simulink model "JLN_Sun_AUV_ver9"  (R2021a)
settings: Solver=VariableStepAuto  StartTime=0.0  StopTime=150  RelTol=1e-3
StopFcn:
  | figure(2)
  | plot3(Position_Data(1,1),Position_Data(1,2),Position_Data(1,3),'r*')
  | hold on
  | plot3(Position_Data(:,1),Position_Data(:,2),Position_Data(:,3));
  | plot3(Position_Data(end,1),Position_Data(end,2),Position_Data(end,3),'g*');
  | grid on
  | legend('Start Point','Trajectory','End Point')
libraries: pid_lib x4, sharedtransform x1
settings Model: Creator=logan  LastModifiedBy=naido
settings DataIOCC: ReturnWorkspaceOutputs=off

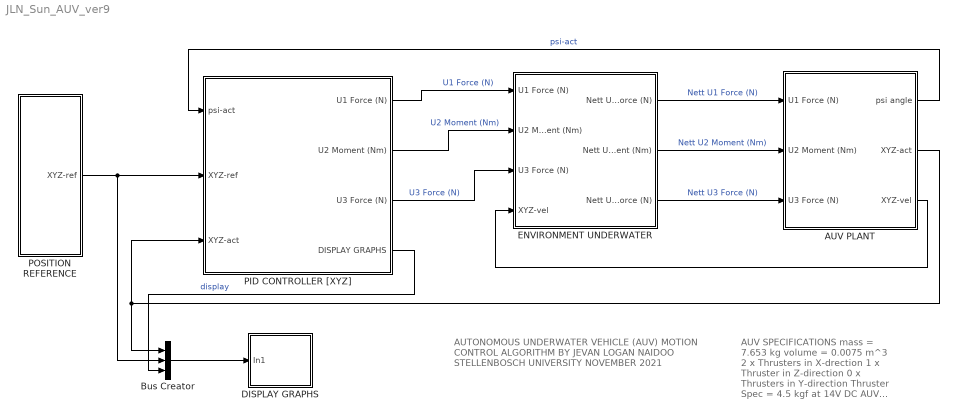
== system JLN_Sun_AUV_ver9 ==
  note: AUV SPECIFICATIONS
      | mass = 7.653 kg
      | volume = 0.0075 m^3
      | 2 x Thrusters in X-drection
      | 1 x Thruster in Z-direction
      | 0 x Thrusters in Y-direction
      | Thruster Spec = 4.5 kgf at 14V DC
      | AUV (LxWxH) = 0.500 x 0.250 x 0.150
  note: AUTONOMOUS UNDERWATER VEHICLE (AUV)
      |
      | MOTION CONTROL ALGORITHM
      | BY JEVAN LOGAN NAIDOO
      | STELLENBOSCH UNIVERSITY
      | NOVEMBER 2021
  AUV PLANT : Subsystem
  Bus Creator : BusCreator  Inputs=3
  DISPLAY GRAPHS : Subsystem
  ENVIRONMENT UNDERWATER : Subsystem
  PID CONTROLLER [XYZ] : Subsystem
  POSITION REFERENCE : Subsystem
  wires:
  AUV PLANT/1(psi angle) -> PID CONTROLLER [XYZ]/1(psi-act)  "psi-act"
  AUV PLANT/2(XYZ-act) -> PID CONTROLLER [XYZ]/3(XYZ-act), Bus Creator/1
  POSITION REFERENCE/1(XYZ-ref) -> Bus Creator/2, PID CONTROLLER [XYZ]/2(XYZ-ref)
  Bus Creator/1 -> DISPLAY GRAPHS/1(In1)
  PID CONTROLLER [XYZ]/4(DISPLAY GRAPHS) -> Bus Creator/3  "display"
  PID CONTROLLER [XYZ]/1(U1 Force (N)) -> ENVIRONMENT UNDERWATER/1(U1 Force (N))  "U1 Force (N)"
  PID CONTROLLER [XYZ]/2(U2 Moment (Nm)) -> ENVIRONMENT UNDERWATER/2(U2 Moment (Nm))  "U2 Moment (Nm)"
  PID CONTROLLER [XYZ]/3(U3 Force (N)) -> ENVIRONMENT UNDERWATER/3(U3 Force (N))  "U3 Force (N)"
  ENVIRONMENT UNDERWATER/1(Nett U1 Force (N)) -> AUV PLANT/1(U1 Force (N))  "Nett U1 Force (N)"
  ENVIRONMENT UNDERWATER/2(Nett U2 Moment (Nm)) -> AUV PLANT/2(U2 Moment (Nm))  "Nett U2 Moment (Nm)"
  ENVIRONMENT UNDERWATER/3(Nett U3 Force (N)) -> AUV PLANT/3(U3 Force (N))  "Nett U3 Force (N)"
  AUV PLANT/3(XYZ-vel) -> ENVIRONMENT UNDERWATER/4(XYZ-vel)

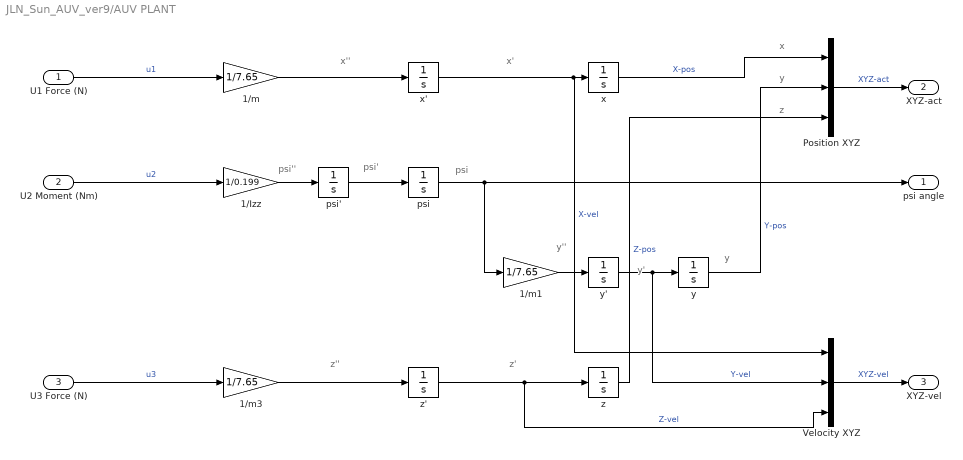
== system JLN_Sun_AUV_ver9/AUV PLANT ==
  note: z''
  note: y
  note: y'
  note: y''
  note: x
  note: psi
  note: psi'
  note: psi''
  note: x''
  note: x'
  note: z'
  note: z
  note: y
  U1 Force (N) : Inport
  U2 Moment (Nm) : Inport  Port=2
  U3 Force (N) : Inport  Port=3
  1/Izz : Gain  Gain=1/0.199
  1/m : Gain  Gain=1/7.65
  1/m1 : Gain  Gain=1/7.65
  1/m3 : Gain  Gain=1/7.65
  Position XYZ : Mux  Inputs=3
  Velocity XYZ : BusCreator  Inputs=3
  psi : Integrator
  psi' : Integrator
  x : Integrator
  x' : Integrator
  y : Integrator
  y' : Integrator
  z : Integrator
  z' : Integrator
  psi angle : Outport
  XYZ-act : Outport  Port=2
  XYZ-vel : Outport  Port=3
  wires:
  x/1 -> Position XYZ/1  "X-pos"
  y/1 -> Position XYZ/2  "Y-pos"
  U1 Force (N)/1 -> 1/m/1  "u1"
  U2 Moment (Nm)/1 -> 1/Izz/1  "u2"
  psi/1 -> 1/m1/1, psi angle/1
  psi'/1 -> psi/1
  1/Izz/1 -> psi'/1
  x'/1 -> Velocity XYZ/1, x/1  "X-vel"
  y'/1 -> Velocity XYZ/2, y/1  "Y-vel"
  1/m/1 -> x'/1
  1/m1/1 -> y'/1
  1/m3/1 -> z'/1
  z'/1 -> Velocity XYZ/3, z/1  "Z-vel"
  z/1 -> Position XYZ/3  "Z-pos"
  U3 Force (N)/1 -> 1/m3/1  "u3"
  Position XYZ/1 -> XYZ-act/1  "XYZ-act"
  Velocity XYZ/1 -> XYZ-vel/1  "XYZ-vel"

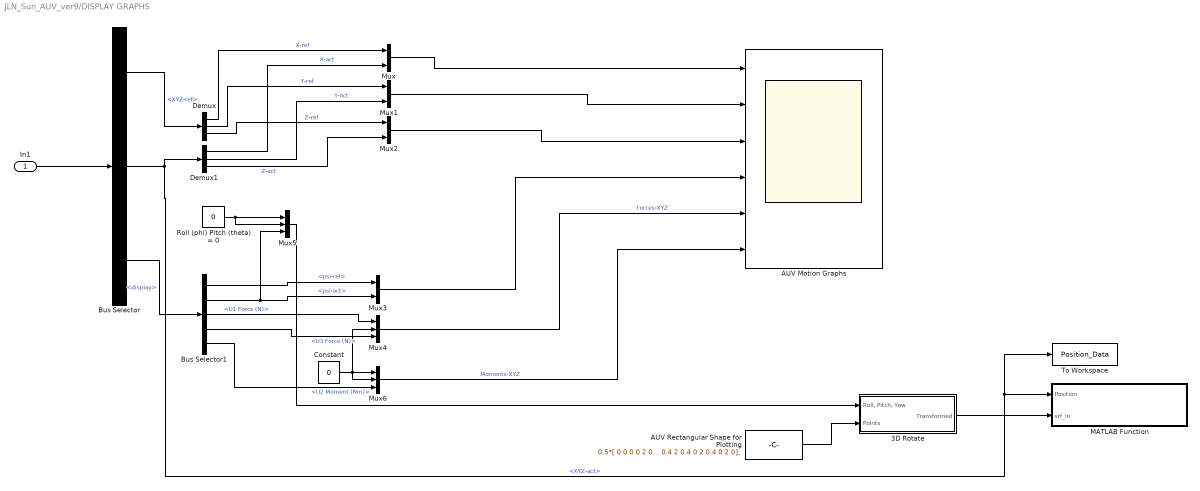
== system JLN_Sun_AUV_ver9/DISPLAY GRAPHS ==
  In1 : Inport
  "3D Rotate " : Subsystem
  AUV Motion Graphs : Scope  NumInputPorts=6
  AUV Rectangular Shape for Plotting : Constant  Value=|
      | 0.5*[	0		0		0
      | 	0		2		0
      | 	0.4		2		0
      | 	0.4		0		0
      | 	0		0		0
      | 	0		0		0.4
      | 	0		2		0.4
      | 	0.4		2		0.4
      | 	0.4		0		0.4
      | 	0		0		0.4
      | 	0.4		0		0.4
      | 	0.4		0		0
      | 	0.4		2		0
      | 	0.4		2		0.4
      | 	0		2		0.4
      | 	0		2		0];
  Bus Selector : BusSelector  OutputSignals=XYZ-ref,XYZ-act,display
  Bus Selector1 : BusSelector  OutputSignals=psi-ref,psi-act,U1 Force (N),U3 Force (N),U2 Moment (Nm)
  Constant : Constant  Value=0
  Demux : Demux  Outputs=3
  Demux1 : Demux  Outputs=3
  MATLAB Function : MATLAB Function  TreatAsAtomicUnit=on  SystemSampleTime=0.05
  Mux{,1..3} (4 alike) : Mux  Inputs=2
  Mux4 : Mux  Inputs=3
  Mux5 : Mux  Inputs=3
  Mux6 : Mux  Inputs=3
  Roll (phi) Pitch (theta) = 0 : Constant  Value=0
  To Workspace : ToWorkspace  VariableName=Position_Data  SampleTime=-1
  wires:
  Mux2/1 -> AUV Motion Graphs/3
  Mux3/1 -> AUV Motion Graphs/4
  In1/1 -> Bus Selector/1
  Mux/1 -> AUV Motion Graphs/1
  Mux1/1 -> AUV Motion Graphs/2
  Roll (phi) Pitch (theta) = 0/1 -> Mux5/1, Mux5/2
  Mux5/1 -> "3D Rotate "/1("Roll, Pitch, Yaw")
  Bus Selector/1 -> Demux/1  "<XYZ-ref>"
  Demux/1 -> Mux/1  "X-ref"
  Demux/2 -> Mux1/1  "Y-ref"
  Demux/3 -> Mux2/1  "Z-ref"
  Bus Selector/2 -> To Workspace/1, MATLAB Function/1(Position), Demux1/1  "<XYZ-act>"
  Demux1/1 -> Mux/2  "X-act"
  Demux1/2 -> Mux1/2  "Y-act"
  Demux1/3 -> Mux2/2  "Z-act"
  Bus Selector/3 -> Bus Selector1/1  "<display>"
  Bus Selector1/1 -> Mux3/1  "<psi-ref>"
  Bus Selector1/2 -> Mux5/3, Mux3/2  "<psi-act>"
  Bus Selector1/3 -> Mux4/1  "<U1 Force (N)>"
  Constant/1 -> Mux4/2, Mux6/2, Mux6/1
  Mux4/1 -> AUV Motion Graphs/5  "Forces-XYZ"
  Bus Selector1/5 -> Mux6/3  "<U2 Moment (Nm)>"
  Mux6/1 -> AUV Motion Graphs/6  "Moments-XYZ"
  Bus Selector1/4 -> Mux4/3  "<U3 Force (N)>"
  AUV Rectangular Shape for Plotting/1 -> "3D Rotate "/2(Points)
  "3D Rotate "/1("Transformed ") -> MATLAB Function/2(srf_in)

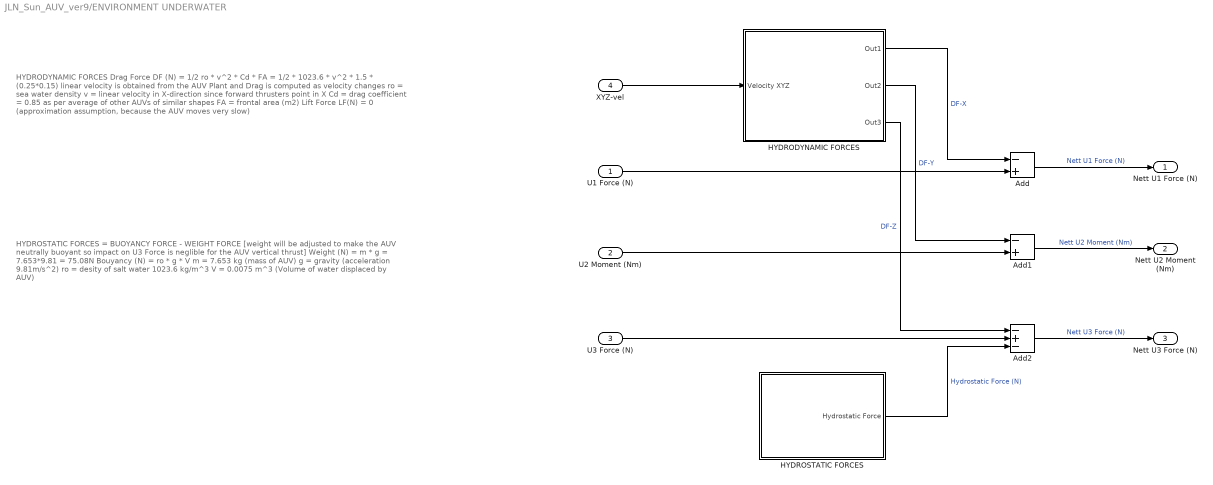
== system JLN_Sun_AUV_ver9/ENVIRONMENT UNDERWATER ==
  note: HYDRODYNAMIC FORCES
      | Drag Force DF (N) = 1/2 ro * v^2 * Cd * FA = 1/2 * 1023.6 * v^2 * 1.5 * (0.25*0.15)
      | linear velocity is obtained from the AUV Plant and Drag is computed as velocity changes
      | ro = sea water density
      | v = linear velocity in X-direction since forward thrusters point in X
      | Cd = drag coefficient = 0.85 as per average of other AUVs of similar shapes
      | FA = frontal area (m2)
      | Lift Force LF(N) = 0 (approximation assumption, because the AUV moves very slow)
  note: HYDROSTATIC FORCES = BUOYANCY FORCE - WEIGHT FORCE
      | [weight will be adjusted to make the AUV neutrally buoyant
      | so impact on U3 Force is neglible for the AUV vertical thrust]
      |
      | Weight (N) = m * g = 7.653*9.81 = 75.08N
      | Bouyancy (N) = ro * g * V
      |
      | m = 7.653 kg (mass of AUV)
      | g = gravity (acceleration 9.81m/s^2)
      | ro = desity of salt water 1023.6 kg/m^3
      | V = 0.0075 m^3 (Volume of water displaced by AUV)
  U1 Force (N) : Inport
  U2 Moment (Nm) : Inport  Port=2
  U3 Force (N) : Inport  Port=3
  XYZ-vel : Inport  Port=4
  Add : Sum  Inputs=-+
  Add1 : Sum  Inputs=-+
  Add2 : Sum  Inputs=-+-
  HYDRODYNAMIC FORCES : Subsystem
  HYDROSTATIC FORCES : Subsystem
  Nett U1 Force (N) : Outport
  Nett U2 Moment (Nm) : Outport  Port=2
  Nett U3 Force (N) : Outport  Port=3
  wires:
  U1 Force (N)/1 -> Add/2
  Add/1 -> Nett U1 Force (N)/1  "Nett U1 Force (N)"
  HYDRODYNAMIC FORCES/1(Out1) -> Add/1  "DF-X"
  XYZ-vel/1 -> HYDRODYNAMIC FORCES/1(Velocity XYZ)
  Add1/1 -> Nett U2 Moment (Nm)/1  "Nett U2 Moment (Nm)"
  U2 Moment (Nm)/1 -> Add1/2
  Add2/1 -> Nett U3 Force (N)/1  "Nett U3 Force (N)"
  U3 Force (N)/1 -> Add2/2
  HYDRODYNAMIC FORCES/2(Out2) -> Add1/1  "DF-Y"
  HYDROSTATIC FORCES/1(Hydrostatic Force) -> Add2/3  "Hydrostatic Force (N)"
  HYDRODYNAMIC FORCES/3(Out3) -> Add2/1  "DF-Z"

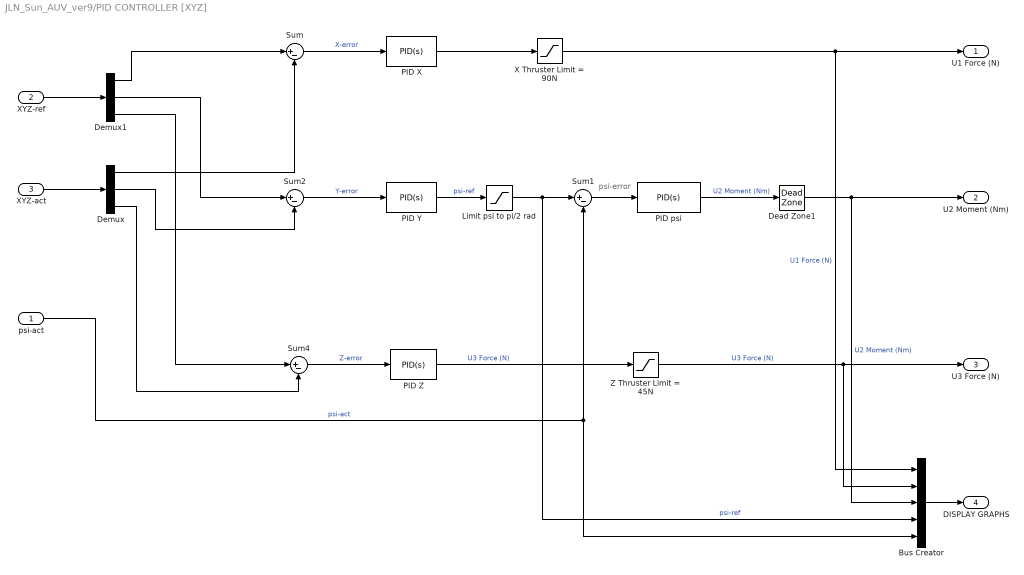
== system JLN_Sun_AUV_ver9/PID CONTROLLER [XYZ] ==
  note: psi-error
  psi-act : Inport
  XYZ-ref : Inport  Port=2
  XYZ-act : Inport  Port=3
  Bus Creator : BusCreator  Inputs=5
  Dead Zone1 : DeadZone  LowerValue=-0.05  UpperValue=0.05  SaturateOnIntegerOverflow=on
  Demux : Demux  Outputs=3
  Demux1 : Demux  Outputs=3
  Limit psi to pi/2 rad : Saturate  UpperLimit=pi/2  LowerLimit=-pi/2
  PID X : pid_lib/PID Controller  Controller=PID  Form=Parallel  TimeDomain=Continuous-time  UseExternalTs=off  SampleTime=-1  IntegratorMethod=Forward Euler  FilterMethod=Forward Euler  ControllerParametersSource=internal  P=8.56108817858543  I=1.15869395657102  D=15.5065166812013  UseFilter=on  N=33.1713932433901  TunerSelectOption=Transfer Function Based (PID Tuner App)  InitialConditionSource=internal  InitialConditionForIntegrator=0  InitialConditionForFilter=0  DifferentiatorICPrevScaledInput=0  ExternalReset=none  TrackingMode=off  Kt=1  LimitOutput=off  SatLimitsSource=internal  UpperSaturationLimit=90  LowerSaturationLimit=-90  LinearizeAsGain=off  AntiWindupMode=none  Kb=1  POutMin=[]  POutMax=[]  IOutMin=[]  IOutMax=[]  DOutMin=[]  DOutMax=[]  NOutMin=[]  NOutMax=[]  SumOutMin=[]  SumOutMax=[]  SaturationOutMin=[]  SaturationOutMax=[]  PParamMin=[]  PParamMax=[]  IParamMin=[]  IParamMax=[]  DParamMin=[]  DParamMax=[]  NParamMin=[]  NParamMax=[]  KbParamMin=[]  KbParamMax=[]  KtParamMin=[]  KtParamMax=[]  KbOutMin=[]  KbOutMax=[]  KtOutMin=[]  KtOutMax=[]  IntegratorOutMin=[]  IntegratorOutMax=[]  FilterOutMin=[]  FilterOutMax=[]  SumI1OutMin=[]  SumI1OutMax=[]  SumI2OutMin=[]  SumI2OutMax=[]  SumI3OutMin=[]  SumI3OutMax=[]  SumI4OutMin=[]  SumI4OutMax=[]  SumDOutMin=[]  SumDOutMax=[]  DifferentiatorOutMin=[]  DifferentiatorOutMax=[]  FilterDiffOutCoefMin=[]  FilterDiffOutCoefMax=[]  ReciprocalOutMin=[]  ReciprocalOutMax=[]  SumDenOutMin=[]  SumDenOutMax=[]  SumNumOutMin=[]  SumNumOutMax=[]  DivideOutMin=[]  DivideOutMax=[]  UdiffTsProdOutMin=[]  UdiffTsProdOutMax=[]  NTsProdOutMin=[]  NTsProdOutMax=[]  UintegralTsProdOutMin=[]  UintegralTsProdOutMax=[]  UngainTsProdOutMin=[]  UngainTsProdOutMax=[]  IntegratorContinuousStateAttributes=''  IntegratorStateMustResolveToSignalObject=off  IntegratorRTWStateStorageClass=Auto  FilterContinuousStateAttributes=''  FilterStateMustResolveToSignalObject=off  FilterRTWStateStorageClass=Auto  ParallelPVariant=InternalParameters  IdealPVariant=Disabled  IVariant=InternalParameters  DVariant=InternalParameters  IntegratorVariant=Continuous  SatVariant=Disabled  AWVariant=Passthrough  PCopyVariant=Disabled  TRVariant=Disabled  FdbkBlocksVariant=Forward  IdealPFdbkVariant=Disabled  SatFdbkVariant=Disabled  DerivativeFilterVariant=ContFilter  NVariant=InternalParameters  NCopyVariant=Disabled  FilterICVariant=InternalICsFilter  IntegratorICVariant=InternalICs  ExternalResetVariant=Disabled  TRSumVariant=Passthrough  SumFdbkVariant=Disabled  SumVariant=Sum_PID  TsampFilterVariant=InternalTs  TsampNgainVariant=Passthrough  TsampIntegralVariant=Passthrough  ExternalSaturationOutDataTypeStr=Inherit: Same as second input
  PID Y : pid_lib/PID Controller  Controller=PID  Form=Parallel  TimeDomain=Continuous-time  UseExternalTs=off  SampleTime=-1  IntegratorMethod=Forward Euler  FilterMethod=Forward Euler  ControllerParametersSource=internal  P=0.5  I=0  D=10  UseFilter=on  N=100  TunerSelectOption=Transfer Function Based (PID Tuner App)  InitialConditionSource=internal  InitialConditionForIntegrator=0  InitialConditionForFilter=0  DifferentiatorICPrevScaledInput=0  ExternalReset=none  TrackingMode=off  Kt=1  LimitOutput=off  SatLimitsSource=internal  UpperSaturationLimit=pi/2  LowerSaturationLimit=-pi/2  LinearizeAsGain=off  AntiWindupMode=none  Kb=1  POutMin=[]  POutMax=[]  IOutMin=[]  IOutMax=[]  DOutMin=[]  DOutMax=[]  NOutMin=[]  NOutMax=[]  SumOutMin=[]  SumOutMax=[]  SaturationOutMin=[]  SaturationOutMax=[]  PParamMin=[]  PParamMax=[]  IParamMin=[]  IParamMax=[]  DParamMin=[]  DParamMax=[]  NParamMin=[]  NParamMax=[]  KbParamMin=[]  KbParamMax=[]  KtParamMin=[]  KtParamMax=[]  KbOutMin=[]  KbOutMax=[]  KtOutMin=[]  KtOutMax=[]  IntegratorOutMin=[]  IntegratorOutMax=[]  FilterOutMin=[]  FilterOutMax=[]  SumI1OutMin=[]  SumI1OutMax=[]  SumI2OutMin=[]  SumI2OutMax=[]  SumI3OutMin=[]  SumI3OutMax=[]  SumI4OutMin=[]  SumI4OutMax=[]  SumDOutMin=[]  SumDOutMax=[]  DifferentiatorOutMin=[]  DifferentiatorOutMax=[]  FilterDiffOutCoefMin=[]  FilterDiffOutCoefMax=[]  ReciprocalOutMin=[]  ReciprocalOutMax=[]  SumDenOutMin=[]  SumDenOutMax=[]  SumNumOutMin=[]  SumNumOutMax=[]  DivideOutMin=[]  DivideOutMax=[]  UdiffTsProdOutMin=[]  UdiffTsProdOutMax=[]  NTsProdOutMin=[]  NTsProdOutMax=[]  UintegralTsProdOutMin=[]  UintegralTsProdOutMax=[]  UngainTsProdOutMin=[]  UngainTsProdOutMax=[]  IntegratorContinuousStateAttributes=''  IntegratorStateMustResolveToSignalObject=off  IntegratorRTWStateStorageClass=Auto  FilterContinuousStateAttributes=''  FilterStateMustResolveToSignalObject=off  FilterRTWStateStorageClass=Auto  ParallelPVariant=InternalParameters  IdealPVariant=Disabled  IVariant=InternalParameters  DVariant=InternalParameters  IntegratorVariant=Continuous  SatVariant=Disabled  AWVariant=Passthrough  PCopyVariant=Disabled  TRVariant=Disabled  FdbkBlocksVariant=Forward  IdealPFdbkVariant=Disabled  SatFdbkVariant=Disabled  DerivativeFilterVariant=ContFilter  NVariant=InternalParameters  NCopyVariant=Disabled  FilterICVariant=InternalICsFilter  IntegratorICVariant=InternalICs  ExternalResetVariant=Disabled  TRSumVariant=Passthrough  SumFdbkVariant=Disabled  SumVariant=Sum_PID  TsampFilterVariant=InternalTs  TsampNgainVariant=Passthrough  TsampIntegralVariant=Passthrough  ExternalSaturationOutDataTypeStr=Inherit: Same as second input
  PID Z : pid_lib/PID Controller  Controller=PID  Form=Parallel  TimeDomain=Continuous-time  UseExternalTs=off  SampleTime=-1  IntegratorMethod=Forward Euler  FilterMethod=Forward Euler  ControllerParametersSource=internal  P=1.42044636402422  I=0.0664978815901045  D=7.45049550922618  UseFilter=on  N=5.45397025421619  TunerSelectOption=Transfer Function Based (PID Tuner App)  InitialConditionSource=internal  InitialConditionForIntegrator=0  InitialConditionForFilter=0  DifferentiatorICPrevScaledInput=0  ExternalReset=none  TrackingMode=off  Kt=1  LimitOutput=off  SatLimitsSource=internal  UpperSaturationLimit=45  LowerSaturationLimit=-45  LinearizeAsGain=on  AntiWindupMode=none  Kb=1  POutMin=[]  POutMax=[]  IOutMin=[]  IOutMax=[]  DOutMin=[]  DOutMax=[]  NOutMin=[]  NOutMax=[]  SumOutMin=[]  SumOutMax=[]  SaturationOutMin=[]  SaturationOutMax=[]  PParamMin=[]  PParamMax=[]  IParamMin=[]  IParamMax=[]  DParamMin=[]  DParamMax=[]  NParamMin=[]  NParamMax=[]  KbParamMin=[]  KbParamMax=[]  KtParamMin=[]  KtParamMax=[]  KbOutMin=[]  KbOutMax=[]  KtOutMin=[]  KtOutMax=[]  IntegratorOutMin=[]  IntegratorOutMax=[]  FilterOutMin=[]  FilterOutMax=[]  SumI1OutMin=[]  SumI1OutMax=[]  SumI2OutMin=[]  SumI2OutMax=[]  SumI3OutMin=[]  SumI3OutMax=[]  SumI4OutMin=[]  SumI4OutMax=[]  SumDOutMin=[]  SumDOutMax=[]  DifferentiatorOutMin=[]  DifferentiatorOutMax=[]  FilterDiffOutCoefMin=[]  FilterDiffOutCoefMax=[]  ReciprocalOutMin=[]  ReciprocalOutMax=[]  SumDenOutMin=[]  SumDenOutMax=[]  SumNumOutMin=[]  SumNumOutMax=[]  DivideOutMin=[]  DivideOutMax=[]  UdiffTsProdOutMin=[]  UdiffTsProdOutMax=[]  NTsProdOutMin=[]  NTsProdOutMax=[]  UintegralTsProdOutMin=[]  UintegralTsProdOutMax=[]  UngainTsProdOutMin=[]  UngainTsProdOutMax=[]  IntegratorContinuousStateAttributes=''  IntegratorStateMustResolveToSignalObject=off  IntegratorRTWStateStorageClass=Auto  FilterContinuousStateAttributes=''  FilterStateMustResolveToSignalObject=off  FilterRTWStateStorageClass=Auto  ParallelPVariant=InternalParameters  IdealPVariant=Disabled  IVariant=InternalParameters  DVariant=InternalParameters  IntegratorVariant=Continuous  SatVariant=Disabled  AWVariant=Passthrough  PCopyVariant=Disabled  TRVariant=Disabled  FdbkBlocksVariant=Forward  IdealPFdbkVariant=Disabled  SatFdbkVariant=Disabled  DerivativeFilterVariant=ContFilter  NVariant=InternalParameters  NCopyVariant=Disabled  FilterICVariant=InternalICsFilter  IntegratorICVariant=InternalICs  ExternalResetVariant=Disabled  TRSumVariant=Passthrough  SumFdbkVariant=Disabled  SumVariant=Sum_PID  TsampFilterVariant=InternalTs  TsampNgainVariant=Passthrough  TsampIntegralVariant=Passthrough  ExternalSaturationOutDataTypeStr=Inherit: Same as second input
  PID psi : pid_lib/PID Controller  Controller=PID  Form=Parallel  TimeDomain=Continuous-time  UseExternalTs=off  SampleTime=-1  IntegratorMethod=Forward Euler  FilterMethod=Forward Euler  ControllerParametersSource=internal  P=100  I=0  D=20  UseFilter=on  N=100  TunerSelectOption=Transfer Function Based (PID Tuner App)  InitialConditionSource=internal  InitialConditionForIntegrator=0  InitialConditionForFilter=0  DifferentiatorICPrevScaledInput=0  ExternalReset=none  TrackingMode=off  Kt=1  LimitOutput=on  SatLimitsSource=internal  UpperSaturationLimit=11  LowerSaturationLimit=-11  LinearizeAsGain=off  AntiWindupMode=none  Kb=1  POutMin=[]  POutMax=[]  IOutMin=[]  IOutMax=[]  DOutMin=[]  DOutMax=[]  NOutMin=[]  NOutMax=[]  SumOutMin=[]  SumOutMax=[]  SaturationOutMin=[]  SaturationOutMax=[]  PParamMin=[]  PParamMax=[]  IParamMin=[]  IParamMax=[]  DParamMin=[]  DParamMax=[]  NParamMin=[]  NParamMax=[]  KbParamMin=[]  KbParamMax=[]  KtParamMin=[]  KtParamMax=[]  KbOutMin=[]  KbOutMax=[]  KtOutMin=[]  KtOutMax=[]  IntegratorOutMin=[]  IntegratorOutMax=[]  FilterOutMin=[]  FilterOutMax=[]  SumI1OutMin=[]  SumI1OutMax=[]  SumI2OutMin=[]  SumI2OutMax=[]  SumI3OutMin=[]  SumI3OutMax=[]  SumI4OutMin=[]  SumI4OutMax=[]  SumDOutMin=[]  SumDOutMax=[]  DifferentiatorOutMin=[]  DifferentiatorOutMax=[]  FilterDiffOutCoefMin=[]  FilterDiffOutCoefMax=[]  ReciprocalOutMin=[]  ReciprocalOutMax=[]  SumDenOutMin=[]  SumDenOutMax=[]  SumNumOutMin=[]  SumNumOutMax=[]  DivideOutMin=[]  DivideOutMax=[]  UdiffTsProdOutMin=[]  UdiffTsProdOutMax=[]  NTsProdOutMin=[]  NTsProdOutMax=[]  UintegralTsProdOutMin=[]  UintegralTsProdOutMax=[]  UngainTsProdOutMin=[]  UngainTsProdOutMax=[]  IntegratorContinuousStateAttributes=''  IntegratorStateMustResolveToSignalObject=off  IntegratorRTWStateStorageClass=Auto  FilterContinuousStateAttributes=''  FilterStateMustResolveToSignalObject=off  FilterRTWStateStorageClass=Auto  ParallelPVariant=InternalParameters  IdealPVariant=Disabled  IVariant=InternalParameters  DVariant=InternalParameters  IntegratorVariant=Continuous  SatVariant=Enabled  AWVariant=Passthrough  PCopyVariant=Disabled  TRVariant=Disabled  FdbkBlocksVariant=Forward  IdealPFdbkVariant=Disabled  SatFdbkVariant=Disabled  DerivativeFilterVariant=ContFilter  NVariant=InternalParameters  NCopyVariant=Disabled  FilterICVariant=InternalICsFilter  IntegratorICVariant=InternalICs  ExternalResetVariant=Disabled  TRSumVariant=Passthrough  SumFdbkVariant=Disabled  SumVariant=Sum_PID  TsampFilterVariant=InternalTs  TsampNgainVariant=Passthrough  TsampIntegralVariant=Passthrough  ExternalSaturationOutDataTypeStr=Inherit: Same as second input
  Sum{,1..2,4} (4 alike) : Sum  Inputs=|+-
  X Thruster Limit = 90N : Saturate  UpperLimit=90  LowerLimit=-90
  Z Thruster Limit = 45N : Saturate  UpperLimit=45  LowerLimit=-45
  U1 Force (N) : Outport
  U2 Moment (Nm) : Outport  Port=2
  U3 Force (N) : Outport  Port=3
  DISPLAY GRAPHS : Outport  Port=4
  wires:
  Demux1/2 -> Sum2/1
  PID Z/1 -> Z Thruster Limit = 45N/1  "U3 Force (N)"
  Demux/2 -> Sum2/2
  Demux1/1 -> Sum/1
  PID Y/1 -> Limit psi to pi/2 rad/1  "psi-ref"
  Sum1/1 -> PID psi/1
  Sum4/1 -> PID Z/1  "Z-error"
  psi-act/1 -> Bus Creator/5, Sum1/2  "psi-act"
  Demux/3 -> Sum4/2
  PID psi/1 -> Dead Zone1/1  "U2 Moment (Nm)"
  Sum/1 -> PID X/1  "X-error"
  Demux/1 -> Sum/2
  PID X/1 -> X Thruster Limit = 90N/1
  Sum2/1 -> PID Y/1  "Y-error"
  Dead Zone1/1 -> U2 Moment (Nm)/1, Bus Creator/3  "U2 Moment (Nm)"
  XYZ-act/1 -> Demux/1
  XYZ-ref/1 -> Demux1/1
  Demux1/3 -> Sum4/1
  Bus Creator/1 -> DISPLAY GRAPHS/1
  Z Thruster Limit = 45N/1 -> U3 Force (N)/1, Bus Creator/2  "U3 Force (N)"
  X Thruster Limit = 90N/1 -> U1 Force (N)/1, Bus Creator/1  "U1 Force (N)"
  Limit psi to pi/2 rad/1 -> Bus Creator/4, Sum1/1  "psi-ref"

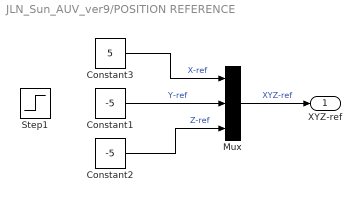
== system JLN_Sun_AUV_ver9/POSITION REFERENCE ==
  Constant1 : Constant  Value=-5
  Constant2 : Constant  Value=-5
  Constant3 : Constant  Value=5
  Mux : Mux  Inputs=3
  Step1 : Step  Time=50  After=-8  SampleTime=0
  XYZ-ref : Outport
  wires:
  Constant3/1 -> Mux/1  "X-ref"
  Constant2/1 -> Mux/3  "Z-ref"
  Mux/1 -> XYZ-ref/1  "XYZ-ref"
  Constant1/1 -> Mux/2  "Y-ref"

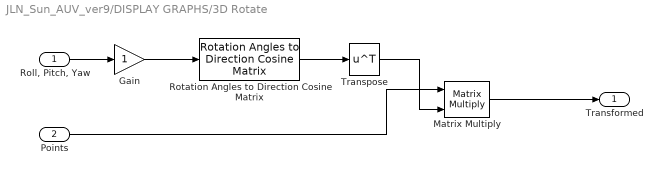
== system JLN_Sun_AUV_ver9/DISPLAY GRAPHS/3D Rotate  ==
  "Roll, Pitch, Yaw" : Inport
  Points : Inport  Port=2
  Gain : Gain
  Matrix Multiply : Product  Multiplication=Matrix(*)
  Rotation Angles to Direction Cosine Matrix : sharedtransform/Rotation Angles to Direction Cosine Matrix  rotationOrder=XYZ  aMode=aMode
      settings: SourceProductBaseCode=AE,PW,DR,MT,UV,VE
  Transpose : Math  Operator=transpose  SignedPower=on  SaturateOnIntegerOverflow=on
  "Transformed " : Outport  VectorParamsAs1DForOutWhenUnconnected=off
  wires:
  Matrix Multiply/1 -> "Transformed "/1
  Rotation Angles to Direction Cosine Matrix/1 -> Transpose/1
  Points/1 -> Matrix Multiply/1
  "Roll, Pitch, Yaw"/1 -> Gain/1
  Transpose/1 -> Matrix Multiply/2
  Gain/1 -> Rotation Angles to Direction Cosine Matrix/1

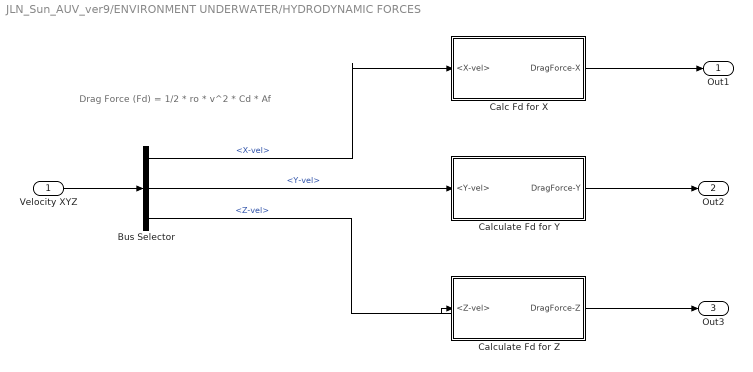
== system JLN_Sun_AUV_ver9/ENVIRONMENT UNDERWATER/HYDRODYNAMIC FORCES ==
  note: Drag Force (Fd) = 1/2 * ro * v^2 * Cd * Af
  Velocity XYZ : Inport
  Bus Selector : BusSelector  OutputSignals=X-vel,Y-vel,Z-vel
  Calc Fd for X : Subsystem
  Calculate Fd for Y : Subsystem
  Calculate Fd for Z : Subsystem
  Out1 : Outport
  Out2 : Outport  Port=2
  Out3 : Outport  Port=3
  wires:
  Velocity XYZ/1 -> Bus Selector/1
  Bus Selector/1 -> Calc Fd for X/1(<X-vel>)  "<X-vel>"
  Calc Fd for X/1(DragForce-X) -> Out1/1
  Bus Selector/2 -> Calculate Fd for Y/1(<Y-vel>)  "<Y-vel>"
  Calculate Fd for Y/1(DragForce-Y) -> Out2/1
  Bus Selector/3 -> Calculate Fd for Z/1(<Z-vel>)  "<Z-vel>"
  Calculate Fd for Z/1(DragForce-Z) -> Out3/1

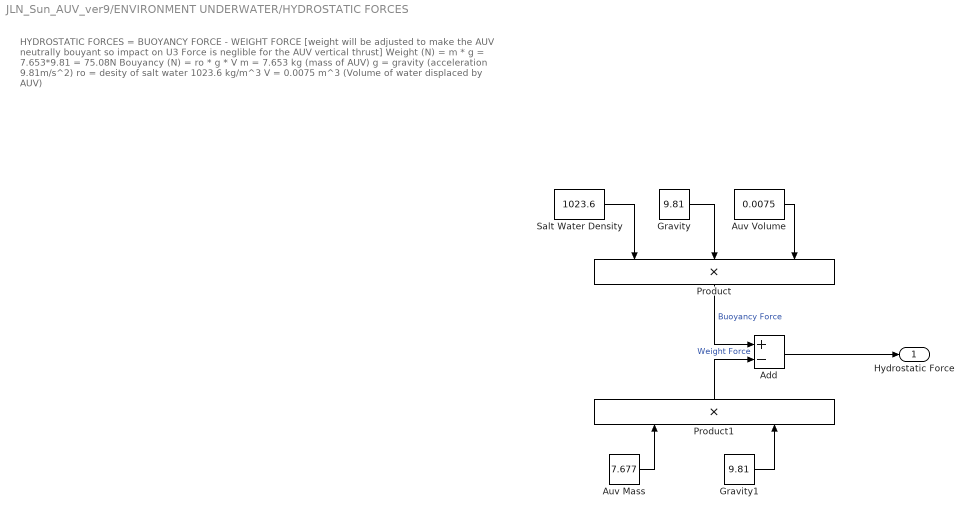
== system JLN_Sun_AUV_ver9/ENVIRONMENT UNDERWATER/HYDROSTATIC FORCES ==
  note: HYDROSTATIC FORCES = BUOYANCY FORCE - WEIGHT FORCE
      | [weight will be adjusted to make the AUV neutrally bouyant
      | so impact on U3 Force is neglible for the AUV vertical thrust]
      |
      | Weight (N) = m * g = 7.653*9.81 = 75.08N
      | Bouyancy (N) = ro * g * V
      |
      | m = 7.653 kg (mass of AUV)
      | g = gravity (acceleration 9.81m/s^2)
      | ro = desity of salt water 1023.6 kg/m^3
      | V = 0.0075 m^3 (Volume of water displaced by AUV)
  Add : Sum  Inputs=+-
  Auv Mass : Constant  Value=7.677
  Auv Volume : Constant  Value=0.0075
  Gravity : Constant  Value=9.81
  Gravity1 : Constant  Value=9.81
  Product : Product  Inputs=3
  Product1 : Product
  Salt Water Density : Constant  Value=1023.6
  Hydrostatic Force : Outport
  wires:
  Salt Water Density/1 -> Product/1
  Gravity/1 -> Product/2
  Auv Volume/1 -> Product/3
  Product/1 -> Add/1  "Buoyancy Force"
  Auv Mass/1 -> Product1/1
  Gravity1/1 -> Product1/2
  Product1/1 -> Add/2  "Weight Force"
  Add/1 -> Hydrostatic Force/1

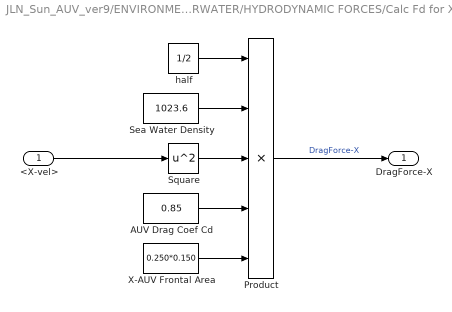
== system JLN_Sun_AUV_ver9/ENVIRONMENT UNDERWATER/HYDRODYNAMIC FORCES/Calc Fd for X ==
  <X-vel> : Inport
  AUV Drag Coef Cd : Constant  Value=0.85
  Product : Product  Inputs=5
  Sea Water Density : Constant  Value=1023.6
  Square : Math  Operator=square  SaturateOnIntegerOverflow=on
  X-AUV Frontal Area : Constant  Value=0.250*0.150
  half : Constant  Value=1/2
  DragForce-X : Outport
  wires:
  X-AUV Frontal Area/1 -> Product/5
  Sea Water Density/1 -> Product/2
  AUV Drag Coef Cd/1 -> Product/4
  Product/1 -> DragForce-X/1  "DragForce-X"
  half/1 -> Product/1
  Square/1 -> Product/3
  <X-vel>/1 -> Square/1

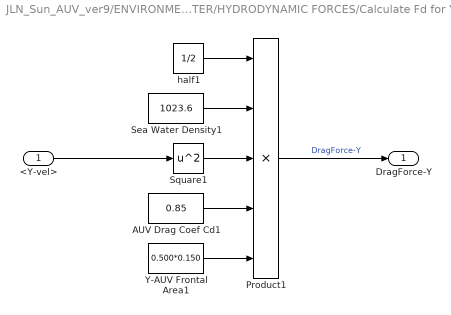
== system JLN_Sun_AUV_ver9/ENVIRONMENT UNDERWATER/HYDRODYNAMIC FORCES/Calculate Fd for Y ==
  <Y-vel> : Inport
  AUV Drag Coef Cd1 : Constant  Value=0.85
  Product1 : Product  Inputs=5
  Sea Water Density1 : Constant  Value=1023.6
  Square1 : Math  Operator=square  SaturateOnIntegerOverflow=on
  Y-AUV Frontal Area1 : Constant  Value=0.500*0.150
  half1 : Constant  Value=1/2
  DragForce-Y : Outport
  wires:
  Product1/1 -> DragForce-Y/1  "DragForce-Y"
  half1/1 -> Product1/1
  Y-AUV Frontal Area1/1 -> Product1/5
  Square1/1 -> Product1/3
  AUV Drag Coef Cd1/1 -> Product1/4
  Sea Water Density1/1 -> Product1/2
  <Y-vel>/1 -> Square1/1

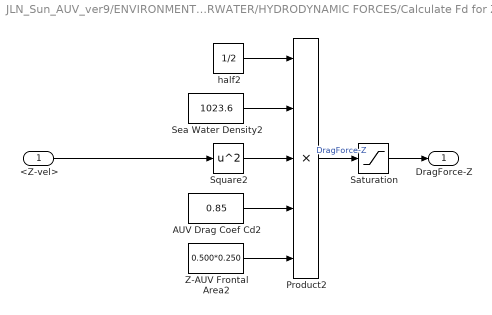
== system JLN_Sun_AUV_ver9/ENVIRONMENT UNDERWATER/HYDRODYNAMIC FORCES/Calculate Fd for Z ==
  <Z-vel> : Inport
  AUV Drag Coef Cd2 : Constant  Value=0.85
  Product2 : Product  Inputs=5
  Saturation : Saturate  UpperLimit=2  LowerLimit=-2  LinearizeAsGain=off
  Sea Water Density2 : Constant  Value=1023.6
  Square2 : Math  Operator=square  SaturateOnIntegerOverflow=on
  Z-AUV Frontal Area2 : Constant  Value=0.500*0.250
  half2 : Constant  Value=1/2
  DragForce-Z : Outport
  wires:
  half2/1 -> Product2/1
  Z-AUV Frontal Area2/1 -> Product2/5
  Sea Water Density2/1 -> Product2/2
  AUV Drag Coef Cd2/1 -> Product2/4
  Square2/1 -> Product2/3
  Product2/1 -> Saturation/1  "DragForce-Z"
  Saturation/1 -> DragForce-Z/1
  <Z-vel>/1 -> Square2/1

== matlab function JLN_Sun_AUV_ver9/DISPLAY GRAPHS/MATLAB Function ==
  data: Position input; srf_in input
function Visualize(Position, srf_in)

    coder.extrinsic('setax'); 
    setax(Position, srf_in);  

end
